simulink model "IM_FluxControllerDesign_vdqsat"  (R2024b)
settings: Solver=VariableStepAuto  StartTime=0.0  StopTime=0.4  RelTol=1e-3
undefined symbols (not defined in the file): ctrl, en, en_d, en_q, im, iSq_step, lambda_Rd_ref, t_iqstep
libraries: cstblocks x3, simulink x2
settings Model: Creator=overflow  LastModifiedBy=matth

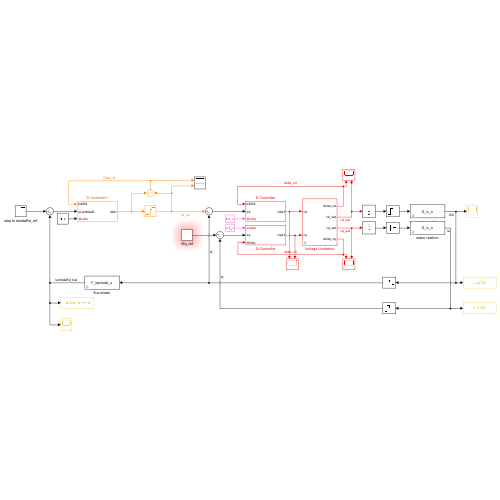
[thumbnail: Simulink's stored preview of the top-level diagram]
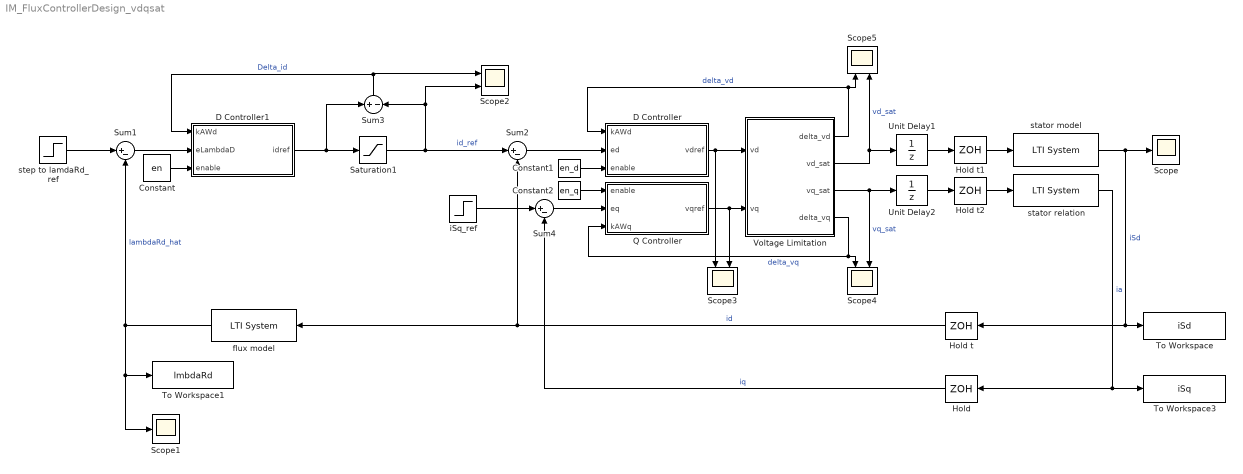
== system IM_FluxControllerDesign_vdqsat ==
  " Hold" : ZeroOrderHold  SampleTime=ctrl.Ts
  " Hold t" : ZeroOrderHold  SampleTime=ctrl.Ts
  " Hold t1" : ZeroOrderHold  SampleTime=ctrl.Ts
  " Hold t2" : ZeroOrderHold  SampleTime=ctrl.Ts
  Constant : Constant  Value=en
  Constant1 : Constant  Value=en_d
  Constant2 : Constant  Value=en_q
  D Controller : Subsystem  mask{Ts=ctrl.Ts, ctrl=ctrl.i}
      mask prompts: Ts "Sampling Time"; ctrl "Controller Struct"
  D Controller1 : Subsystem  mask{Ts=ctrl.Ts, ctrl=ctrl.lambdar}
      mask prompts: Ts "Sampling Time"; ctrl "Controller Struct"
  Q Controller : Subsystem  mask{Ts=ctrl.Ts, ctrl=ctrl.i}
      mask prompts: Ts "Sampling Time"; ctrl "Controller Struct"
  Saturation1 : Saturate  UpperLimit=im.iSmax  LowerLimit=0
  Scope : Scope
  Scope1 : Scope
  Scope{2..5} (4 alike) : Scope  NumInputPorts=2
  Sum1 : Sum  Inputs=|+-
  Sum2 : Sum  Inputs=|+-
  Sum3 : Sum  Inputs=+|-
  Sum4 : Sum  Inputs=|+-
  To Workspace : ToWorkspace  VariableName=iSd  SaveFormat=Timeseries  SampleTime=-1
  To Workspace1 : ToWorkspace  VariableName=lmbdaRd  SaveFormat=Timeseries  SampleTime=-1
  To Workspace3 : ToWorkspace  VariableName=iSq  SaveFormat=Timeseries  SampleTime=-1
  Unit Delay1 : UnitDelay  SampleTime=ctrl.Ts  HasFrameUpgradeWarning=on
  Unit Delay2 : UnitDelay  SampleTime=ctrl.Ts  HasFrameUpgradeWarning=on
  Voltage Limitation : Subsystem  mask{Vmax=im.vSmax}
      mask prompts: Vmax "Max Voltage"
  flux model : cstblocks/LTI System  sys=F_lambdai_z  IC=[0]  PadeOrder=0
  iSq_ref : Step  Time=0  Before=t_iqstep  After=iSq_step  SampleTime=0
  "stator model " : cstblocks/LTI System  sys=G_iv_s  IC=[0]  PadeOrder=0
  stator relation : cstblocks/LTI System  sys=G_iv_s  IC=[0]  PadeOrder=0
  step to lamdaRd_ref : Step  Time=0  After=lambda_Rd_ref  SampleTime=0
  wires:
  Sum1/1 -> D Controller1/2(eLambdaD)
  flux model/1 -> Sum1/2, To Workspace1/1, Scope1/1  "lambdaRd_hat"
  " Hold t"/1 -> Sum2/2, flux model/1  "id"
  " Hold t1"/1 -> "stator model "/1
  "stator model "/1 -> Scope/1, " Hold t"/1, To Workspace/1  "iSd"
  Unit Delay1/1 -> " Hold t1"/1
  step to lamdaRd_ref/1 -> Sum1/1
  Saturation1/1 -> Sum2/1, Scope2/2, Sum3/2  "id_ref"
  D Controller1/1(idref) -> Saturation1/1, Sum3/1
  Sum3/1 -> Scope2/1, D Controller1/1(kAWd)  "Delta_id"
  Constant/1 -> D Controller1/3(enable)
  Constant2/1 -> Q Controller/1(enable)
  Constant1/1 -> D Controller/3(enable)
  Voltage Limitation/3(vq_sat) -> Unit Delay2/1, Scope4/2  "vq_sat"
  Voltage Limitation/4(delta_vq) -> Q Controller/3(kAWq), Scope4/1  "delta_vq"
  Q Controller/1(vqref) -> Scope3/2, Voltage Limitation/2("vq ")
  Voltage Limitation/1(delta_vd) -> Scope5/1, D Controller/1(kAWd)  "delta_vd"
  Sum2/1 -> D Controller/2(ed)
  Voltage Limitation/2(vd_sat) -> Unit Delay1/1, Scope5/2  "vd_sat"
  D Controller/1(vdref) -> Scope3/1, Voltage Limitation/1(vd)
  Unit Delay2/1 -> " Hold t2"/1
  " Hold t2"/1 -> stator relation/1
  stator relation/1 -> " Hold"/1, To Workspace3/1  "ia"
  Sum4/1 -> Q Controller/2(eq)
  " Hold"/1 -> Sum4/2  "iq"
  iSq_ref/1 -> Sum4/1

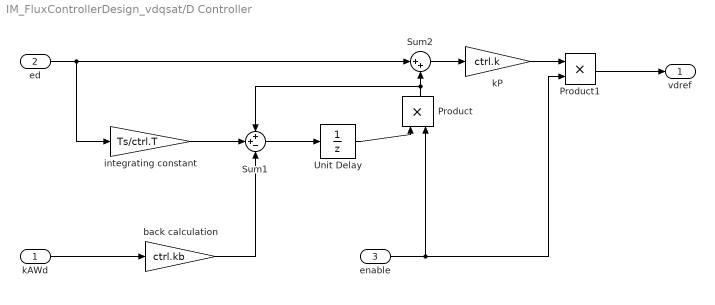
== system IM_FluxControllerDesign_vdqsat/D Controller ==
  kAWd : Inport
  ed : Inport  Port=2
  enable : Inport  Port=3
  Product : Product
  Product1 : Product
  Sum1 : Sum  Inputs=++-
  Sum2 : Sum  Inputs=|++
  Unit Delay : UnitDelay  SampleTime=-1  HasFrameUpgradeWarning=on
  back calculation : Gain  Gain=ctrl.kb
  integrating constant : Gain  Gain=Ts/ctrl.T
  kP : Gain  Gain=ctrl.k
  vdref : Outport
  wires:
  ed/1 -> integrating constant/1, Sum2/1
  Sum2/1 -> kP/1
  kAWd/1 -> back calculation/1
  Sum1/1 -> Unit Delay/1
  Unit Delay/1 -> Product/1
  Product/1 -> Sum1/1, Sum2/2
  kP/1 -> Product1/1
  Product1/1 -> vdref/1
  enable/1 -> Product1/2, Product/2
  integrating constant/1 -> Sum1/2
  back calculation/1 -> Sum1/3

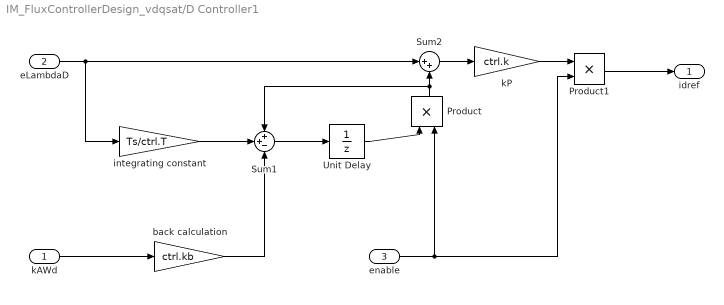
== system IM_FluxControllerDesign_vdqsat/D Controller1 ==
  kAWd : Inport
  eLambdaD : Inport  Port=2
  enable : Inport  Port=3
  Product : Product
  Product1 : Product
  Sum1 : Sum  Inputs=++-
  Sum2 : Sum  Inputs=|++
  Unit Delay : UnitDelay  SampleTime=-1  HasFrameUpgradeWarning=on
  back calculation : Gain  Gain=ctrl.kb
  integrating constant : Gain  Gain=Ts/ctrl.T
  kP : Gain  Gain=ctrl.k
  idref : Outport
  wires:
  eLambdaD/1 -> integrating constant/1, Sum2/1
  Sum2/1 -> kP/1
  kAWd/1 -> back calculation/1
  Sum1/1 -> Unit Delay/1
  Unit Delay/1 -> Product/1
  Product/1 -> Sum1/1, Sum2/2
  kP/1 -> Product1/1
  Product1/1 -> idref/1
  enable/1 -> Product1/2, Product/2
  integrating constant/1 -> Sum1/2
  back calculation/1 -> Sum1/3

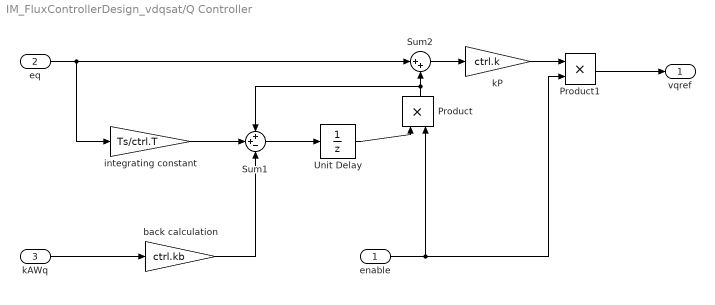
== system IM_FluxControllerDesign_vdqsat/Q Controller ==
  enable : Inport
  eq : Inport  Port=2
  kAWq : Inport  Port=3
  Product : Product
  Product1 : Product
  Sum1 : Sum  Inputs=++-
  Sum2 : Sum  Inputs=|++
  Unit Delay : UnitDelay  SampleTime=-1  HasFrameUpgradeWarning=on
  back calculation : Gain  Gain=ctrl.kb
  integrating constant : Gain  Gain=Ts/ctrl.T
  kP : Gain  Gain=ctrl.k
  vqref : Outport
  wires:
  eq/1 -> integrating constant/1, Sum2/1
  Sum2/1 -> kP/1
  kAWq/1 -> back calculation/1
  Sum1/1 -> Unit Delay/1
  Unit Delay/1 -> Product/1
  Product/1 -> Sum1/1, Sum2/2
  kP/1 -> Product1/1
  Product1/1 -> vqref/1
  enable/1 -> Product1/2, Product/2
  integrating constant/1 -> Sum1/2
  back calculation/1 -> Sum1/3

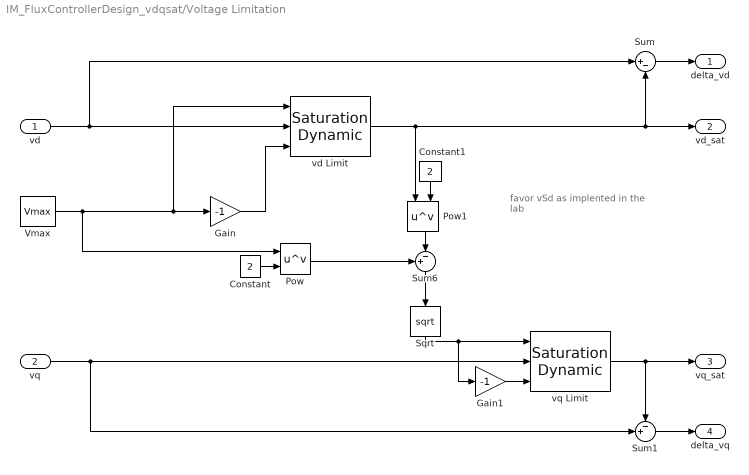
== system IM_FluxControllerDesign_vdqsat/Voltage Limitation ==
  note: favor vSd as implented in the lab
  vd : Inport
  "vq " : Inport  Port=2
  Constant : Constant  Value=2
  Constant1 : Constant  Value=2
  Gain : Gain  Gain=-1
  Gain1 : Gain  Gain=-1
  Pow : Math  Operator=pow  RndMeth=Zero
  Pow1 : Math  Operator=pow  RndMeth=Zero
  Sqrt : Sqrt
  Sum : Sum  Inputs=|+-
  Sum1 : Sum  Inputs=-+|
  Sum6 : Sum  Inputs=+-|
  Vmax : Constant  Value=Vmax
  vd Limit : simulink/Discontinuities/Saturation Dynamic  OutMin=[]  OutMax=[]  OutDataTypeStr=Inherit: Same as second input  OutDataType=fixdt(1, 16)  OutScaling=2^-10  DoSatur=off
  vq Limit : simulink/Discontinuities/Saturation Dynamic  OutMin=[]  OutMax=[]  OutDataTypeStr=Inherit: Same as second input  OutDataType=fixdt(1, 16)  OutScaling=2^-10  DoSatur=off
  delta_vd : Outport  VectorParamsAs1DForOutWhenUnconnected=off
  vd_sat : Outport  Port=2  VectorParamsAs1DForOutWhenUnconnected=off
  vq_sat : Outport  Port=3  VectorParamsAs1DForOutWhenUnconnected=off
  delta_vq : Outport  Port=4  VectorParamsAs1DForOutWhenUnconnected=off
  wires:
  Gain/1 -> vd Limit/3
  vd Limit/1 -> Sum/2, vd_sat/1, Pow1/1
  Sqrt/1 -> Gain1/1, vq Limit/1
  vq Limit/1 -> Sum1/1, vq_sat/1
  Pow/1 -> Sum6/1
  vd/1 -> Sum/1, vd Limit/2
  Sum6/1 -> Sqrt/1
  "vq "/1 -> vq Limit/2, Sum1/2
  Pow1/1 -> Sum6/2
  Vmax/1 -> Pow/1, Gain/1, vd Limit/1
  Gain1/1 -> vq Limit/3
  Sum/1 -> delta_vd/1
  Sum1/1 -> delta_vq/1
  Constant/1 -> Pow/2
  Constant1/1 -> Pow1/2
